simulink model "COM_ViconController_x4morf_quat_withRecov_posMod"  (Simulink 8.6)
settings: Solver=FixedStepDiscrete  StartTime=0.0  StopTime=inf  FixedStep=ComMinSampleTime  RelTol=1e-3
values from neighbouring files (symbols this model uses):
  a_PWM = (MaxThrottle-MinThrottle)/(omega_r_max-omega_r_min)    [RobotParameters.m]
  b_PWM = MinThrottle - a_PWM*omega_r_min    [RobotParameters.m]
  BiasAcc = [-0.0791 0.072 -0.1481]    [AccCalib_Transformation_X4morf_Robot.mat]
  ComMinSampleTime = 1/400    (= 0.0025)    [init_ViconController_x4morf_quat_withRecov_posMod.m]
  dc_close = 25    [RobotParameters.m]
  dc_open = 63    [RobotParameters.m]
  g = 9.81    [RobotParameters.m]    (also in init_ViconController_x4morf_quat_withRecov_posMod.m)
  gamma_max = 89    [RobotParameters.m]
  LandingHeight = 0.08    [init_ViconController_x4morf_quat_withRecov_posMod.m]
  m = 0.380    (= 0.38)    [RobotParameters.m]
  MaxThrottle = 2000    [RobotParameters.m]
  MinThrottle = 1200    [RobotParameters.m]
  PositionSecuMax = [5.5 ; 3 ; 4]    [RobotParameters.m]
  PositionSecuMin = [-0.5; -3; -0.07]    [RobotParameters.m]
  Tacc = [0.9812  -0.03737  -0.0078; 0.0368  0.9984  -0.0083; 0.0232  -0.0002  0.9804]    [AccCalib_Transformation_X4morf_Robot.mat]
  time_unfolding = 230e-3    (= 0.23)    [RobotParameters.m]
  Tmax = .1643    (= 0.1643)    [RobotParameters.m]
  Tmin = .0183    (= 0.0183)    [RobotParameters.m]
  TorquesSat = zeros(3,181)    [gen_iGamma.m]
  Ts_AttitudeLoop = 1/200    (= 0.005)    [init_ViconController_x4morf_quat_withRecov_posMod.m]
  Ts_PositionLoop = 1/100    (= 0.01)    [init_ViconController_x4morf_quat_withRecov_posMod.m]
  Velocity_0 = [Vx_0 Vy_0 Vz_0]    [RobotParameters.m]
undefined symbols (not defined in the file or in its folder): DiscIntNeverNeededParam, Gumstix, MPU6050, UAVstruct
undefined symbols (not defined in the file): AccMax, AccMaxScenario, AccMin, AccMinScenario, b_est0, PositionMax, PositionMin, SpeedMax, SpeedMaxScenario, SpeedMin, SpeedMinScenario, Ts_Wifi
libraries: simulink x40, simulink_extras x11
(part 2 of 3)

== system COM_ViconController_x4morf_quat_withRecov_posMod/GUMSTIX/Torques  Disturbances ==
  Torques : Inport
  Dist_Torques : Inport  Port=2
  " " : Constant  Value=[0 0 0]  OutDataTypeStr=Inherit: Inherit via back propagation
  Add : Sum
  Add1 : Sum
  Add2 : Sum
  Compare To Constant : simulink/Logic and Bit Operations/Compare To Constant  relop===  const=1  OutDataTypeStr=boolean
  Compare To Constant1 : simulink/Logic and Bit Operations/Compare To Constant  relop===  const=3  OutDataTypeStr=boolean
  Demux2 : Demux  Outputs=3
  Demux3 : Demux  Outputs=3
  Multiport Switch : MultiPortSwitch  DataPortForDefault=Additional data port
  Mux : Mux  Inputs=3
  Mux1 : Mux  Inputs=3
  Selector : Selector  InputPortWidth=5  IndexOptions=Index vector (dialog)  Indices=[1 2 3]  OutputSizes=1
  Selector2 : Selector  InputPortWidth=5  IndexOptions=Index vector (dialog)  Indices=4  OutputSizes=1
  Selector3 : Selector  InputPortWidth=5  IndexOptions=Index vector (dialog)  Indices=5  OutputSizes=1
  Triggered Subsystem : Subsystem  TreatAsAtomicUnit=on
  Triggered Subsystem1 : Subsystem  TreatAsAtomicUnit=on
  Torques_Out : Outport
  dist_torques_OUT : Outport  Port=2
  wires:
  Dist_Torques/1 -> Selector2/1, Selector3/1, Selector/1
  Selector/1 -> Triggered Subsystem1/1(TorquesDist Mag), Multiport Switch/3, Triggered Subsystem/1(TorquesDist Mag)
  Selector3/1 -> Mux1/3, Multiport Switch/1, Compare To Constant1/1, Compare To Constant/1
  Demux2/1 -> Add/1
  Demux2/2 -> Add1/1
  Demux2/3 -> Add2/1
  Add/1 -> Mux/1
  Add1/1 -> Mux/2
  Add2/1 -> Mux/3
  Demux3/2 -> Add1/2
  Demux3/1 -> Add/2
  Demux3/3 -> Add2/2
  Selector2/1 -> Mux1/2, Triggered Subsystem1/2(Dt), Triggered Subsystem/2(Dt)
  Torques/1 -> Demux2/1
  Mux/1 -> Torques_Out/1
  Compare To Constant/1 -> Triggered Subsystem/Enable
  Triggered Subsystem/1(DisturbTorques) -> Multiport Switch/2
  Multiport Switch/1 -> Demux3/1, Mux1/1
  " "/1 -> Multiport Switch/5
  Compare To Constant1/1 -> Triggered Subsystem1/Enable
  Triggered Subsystem1/1(DisturbTorques) -> Multiport Switch/4
  Mux1/1 -> dist_torques_OUT/1

== system COM_ViconController_x4morf_quat_withRecov_posMod/GUMSTIX/Torques saturation ==
  Torques : Inport
  gamma [deg] : Inport  Port=2
  Constant : Constant  Value=TorquesSat
  Convert : DataTypeConversion  RndMeth=Nearest
  Demux : Demux  Outputs=3
  Demux1 : Demux  Outputs=3
  Gain : Gain  Gain=-1
  Gain1 : Gain  Gain=-1
  Gain2 : Gain  Gain=-1
  MATLAB Function : MATLAB Function  TreatAsAtomicUnit=on
  Mux4 : Mux  Inputs=3
  Saturation Dynamic : simulink/Discontinuities/Saturation Dynamic  OutMin=[]  OutMax=[]  OutDataTypeStr=Inherit: Same as second input  OutDataType=fixdt(1, 16)  OutScaling=2^-10  DoSatur=off
  Saturation Dynamic1 : simulink/Discontinuities/Saturation Dynamic  OutMin=[]  OutMax=[]  OutDataTypeStr=Inherit: Same as second input  OutDataType=fixdt(1, 16)  OutScaling=2^-10  DoSatur=off
  Saturation Dynamic2 : simulink/Discontinuities/Saturation Dynamic  OutMin=[]  OutMax=[]  OutDataTypeStr=Inherit: Same as second input  OutDataType=fixdt(1, 16)  OutScaling=2^-10  DoSatur=off
  Torques_Sat : Outport
  Sats : Outport  Port=2
  wires:
  Mux4/1 -> Convert/1
  gamma [deg]/1 -> MATLAB Function/2(gamma)
  Constant/1 -> MATLAB Function/1(TorquesSat)
  Demux/1 -> Saturation Dynamic/2
  Demux/2 -> Saturation Dynamic1/2
  Demux/3 -> Saturation Dynamic2/2
  Saturation Dynamic/1 -> Mux4/1
  Saturation Dynamic1/1 -> Mux4/2
  Saturation Dynamic2/1 -> Mux4/3
  Torques/1 -> Demux/1
  Demux1/1 -> Gain/1, Saturation Dynamic/1
  Demux1/2 -> Gain1/1, Saturation Dynamic1/1
  Demux1/3 -> Gain2/1, Saturation Dynamic2/1
  Gain/1 -> Saturation Dynamic/3
  Gain1/1 -> Saturation Dynamic1/3
  Gain2/1 -> Saturation Dynamic2/3
  MATLAB Function/1(TSat) -> Sats/1, Demux1/1
  Convert/1 -> Torques_Sat/1

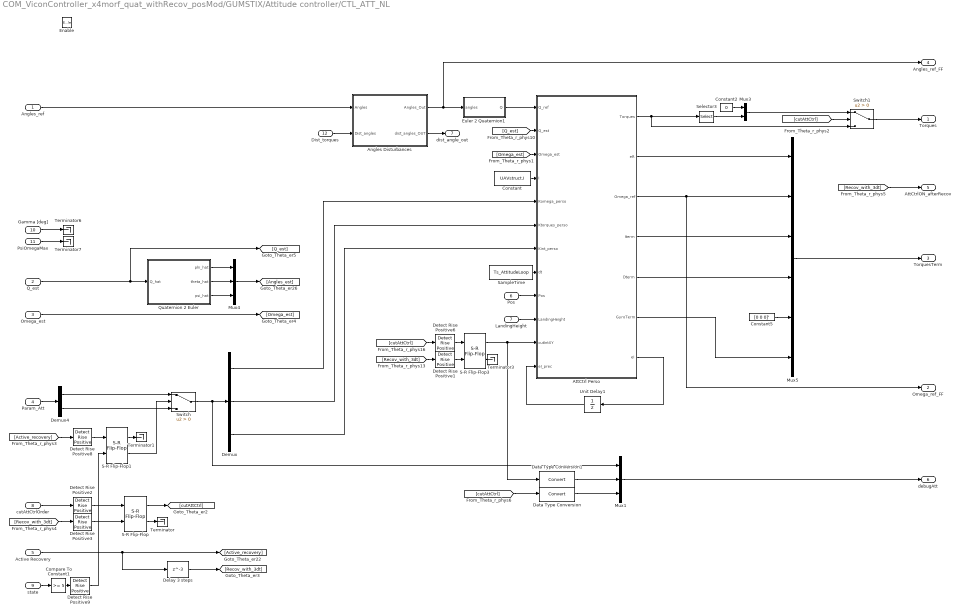
== system COM_ViconController_x4morf_quat_withRecov_posMod/GUMSTIX/Attitude controller/CTL_ATT_NL ==
  Angles_ref : Inport
  Q_est : Inport  Port=2
  Omega_est : Inport  Port=3
  Param_Att : Inport  Port=4
  Active Recovery : Inport  Port=5
  Pos : Inport  Port=6
  LandingHeight : Inport  Port=7
  cutAttCtrlOrder : Inport  Port=8
  state : Inport  Port=9
  Gamma [deg] : Inport  Port=10
  PsiOmegaMax : Inport  Port=11
  Dist_torques : Inport  Port=12
  Enable : EnablePort  StatesWhenEnabling=reset
  Angles Disturbances : Subsystem
  AttCtrl Perso : MATLAB Function  TreatAsAtomicUnit=on
  Compare To Constant1 : simulink/Logic and Bit Operations/Compare To Constant  relop=>=  const=5  OutDataTypeStr=boolean
  Constant : Constant  Value=UAVstruct.I  OutDataTypeStr=Inherit: Inherit via back propagation
  Constant2 : Constant  Value=0  OutDataTypeStr=Inherit: Inherit via back propagation
  Constant5 : Constant  Value=[0 0 0]'  OutDataTypeStr=Inherit: Inherit via back propagation
  Data Type Conversion : DataTypeConversion
  Data Type Conversion1 : DataTypeConversion
  Delay 3 steps : Delay  DelayLength=3  InitialCondition=0
  Demux : Demux  Outputs=[3 3 3]
  Demux4 : Demux  Outputs=2
  Detect Rise Positive{1..3,6,8..9} (6 alike) : simulink/Logic and Bit Operations/Detect Rise Positive  vinit=1  InputProcessing=Inherited  OutDataTypeStr=boolean
  Euler 2 Quaternion1 : MATLAB Function  TreatAsAtomicUnit=on
  Mux1 : Mux  Inputs=[9 1 1]
  Mux3 : Mux  Inputs=[1 2]
  Mux4 : Mux  Inputs=3
  Mux5 : Mux  Inputs=[3 3 3 3 3 3]
  Quaternion 2 Euler : MATLAB Function  TreatAsAtomicUnit=on
  S-R Flip-Flop : simulink_extras/Flip Flops/S-R Flip-Flop  initial_condition=0
  S-R Flip-Flop1 : simulink_extras/Flip Flops/S-R Flip-Flop  initial_condition=0
  S-R Flip-Flop3 : simulink_extras/Flip Flops/S-R Flip-Flop  initial_condition=0
  SampleTime : Constant  Value=Ts_AttitudeLoop  OutDataTypeStr=single  SampleTime=-1
  Selector3 : Selector  InputPortWidth=3  IndexOptions=Index vector (dialog)  Indices=[2 3]  OutputSizes=1
  Switch : Switch  Criteria=u2 > Threshold
  Switch1 : Switch  Criteria=u2 > Threshold
  Terminator{,1,3,6..7} (5 alike) : Terminator
  Unit Delay1 : UnitDelay  InitialCondition=single([0 0 0])  SampleTime=-1
  Torques : Outport  InitialOutput=[0; 0; 0]
  Omega_ref_FF : Outport  Port=2  InitialOutput=[0; 0; 0]
  TorquesTerm : Outport  Port=3  InitialOutput=zeros(18, 1)
  Angles_ref_FF : Outport  Port=4  InitialOutput=[0; 0; 0]
  AttCtrlON_afterRecov : Outport  Port=5  InitialOutput=0
  debugAtt : Outport  Port=6  InitialOutput=zeros(11,0)
  dist_angle_out : Outport  Port=7  InitialOutput=[0; 0; 0; 0; 0]
  wires:
  Constant2/1 -> Mux3/1
  Mux3/1 -> Switch1/1
  [cutAttCtrl] -> Switch1/2
  Active Recovery/1 -> Delay 3 steps/1, [Active_recovery]
  Delay 3 steps/1 -> [Recov_with_3dt]
  [Recov_with_3dt] -> Detect Rise Positive3/1
  [Recov_with_3dt] -> AttCtrlON_afterRecov/1
  Q_est/1 -> [Q_est], Quaternion 2 Euler/1(Q_hat)
  Omega_est/1 -> [Omega_est]
  Quaternion 2 Euler/1(phi_hat) -> Mux4/1
  Quaternion 2 Euler/2(theta_hat) -> Mux4/2
  Quaternion 2 Euler/3(psi_hat) -> Mux4/3
  Mux4/1 -> [Angles_est]
  cutAttCtrlOrder/1 -> Detect Rise Positive2/1
  S-R Flip-Flop/1 -> [cutAttCtrl]
  S-R Flip-Flop/2 -> Terminator/1
  Detect Rise Positive2/1 -> S-R Flip-Flop/1
  Detect Rise Positive3/1 -> S-R Flip-Flop/2
  Demux/1 -> AttCtrl Perso/5(Komega_perso)
  Demux/2 -> AttCtrl Perso/6(Ktorques_perso)
  Euler 2 Quaternion1/1(Q) -> AttCtrl Perso/1(Q_ref)
  AttCtrl Perso/1(Torques) -> Switch1/3, Selector3/1
  AttCtrl Perso/2(eR) -> Mux5/1
  AttCtrl Perso/6(GyroTerm) -> Mux5/6
  Mux5/1 -> TorquesTerm/1
  AttCtrl Perso/3(Omega_ref) -> Omega_ref_FF/1, Mux5/2
  AttCtrl Perso/7(eI) -> Unit Delay1/1
  Unit Delay1/1 -> AttCtrl Perso/12(eI_prec)
  AttCtrl Perso/4(Iterm) -> Mux5/3
  Demux/3 -> AttCtrl Perso/7(Kint_perso)
  Switch1/1 -> Torques/1
  state/1 -> Compare To Constant1/1
  AttCtrl Perso/5(Dterm) -> Mux5/4
  S-R Flip-Flop3/1 -> Data Type Conversion1/1, AttCtrl Perso/11(cutIntXY)
  S-R Flip-Flop3/2 -> Terminator3/1
  [cutAttCtrl] -> Detect Rise Positive6/1
  Detect Rise Positive6/1 -> S-R Flip-Flop3/1
  Detect Rise Positive1/1 -> S-R Flip-Flop3/2
  Gamma [deg]/1 -> Terminator6/1
  PsiOmegaMax/1 -> Terminator7/1
  Constant5/1 -> Mux5/5
  [Recov_with_3dt] -> Detect Rise Positive1/1
  Constant/1 -> AttCtrl Perso/4(I)
  SampleTime/1 -> AttCtrl Perso/8(dt)
  Pos/1 -> AttCtrl Perso/9(Pos)
  LandingHeight/1 -> AttCtrl Perso/10(LandingHeight)
  [Omega_est] -> AttCtrl Perso/3(Omega_est)
  Param_Att/1 -> Demux4/1
  Demux4/1 -> Switch/1
  Demux4/2 -> Switch/3
  Switch/1 -> Mux1/1, Demux/1
  [Active_recovery] -> Detect Rise Positive8/1
  Detect Rise Positive8/1 -> S-R Flip-Flop1/1
  S-R Flip-Flop1/1 -> Terminator1/1
  S-R Flip-Flop1/2 -> Switch/2
  Compare To Constant1/1 -> Detect Rise Positive9/1
  Detect Rise Positive9/1 -> S-R Flip-Flop1/2
  [cutAttCtrl] -> Data Type Conversion/1
  Mux1/1 -> debugAtt/1
  Data Type Conversion/1 -> Mux1/3
  Data Type Conversion1/1 -> Mux1/2
  Angles Disturbances/1(Angles_Out) -> Angles_ref_FF/1, Euler 2 Quaternion1/1(angles)
  Angles Disturbances/2(dist_angles_OUT) -> dist_angle_out/1
  Dist_torques/1 -> Angles Disturbances/2(Dist_angles)
  [Q_est] -> AttCtrl Perso/2(Q_est)
  Angles_ref/1 -> Angles Disturbances/1(Angles)
  Selector3/1 -> Mux3/2

== system COM_ViconController_x4morf_quat_withRecov_posMod/GUMSTIX/Control Mix/Control_mix ==
  Thrust : Inport
  Torques : Inport  Port=2
  gamma [deg] : Inport  Port=3
  Constant : Constant  Value=UAVstruct.iGamma  OutDataTypeStr=Inherit: Inherit via back propagation
  Demux : Demux
  Mixage : MATLAB Function  TreatAsAtomicUnit=on
  Mux1 : Mux  Inputs=2
  Rate Transition : RateTransition
  Saturation1 : Saturate  UpperLimit=inf  LowerLimit=0
  Sqrt1 : Sqrt  SaturateOnIntegerOverflow=on
  omega_r1_ref : Outport
  omega_r2_ref : Outport  Port=2
  omega_r3_ref : Outport  Port=3
  omega_r4_ref : Outport  Port=4
  wires:
  Demux/1 -> omega_r1_ref/1
  Demux/2 -> omega_r2_ref/1
  Demux/3 -> omega_r3_ref/1
  Demux/4 -> omega_r4_ref/1
  Sqrt1/1 -> Rate Transition/1
  Rate Transition/1 -> Demux/1
  Thrust/1 -> Mux1/1
  Torques/1 -> Mux1/2
  Mixage/1(omega2) -> Saturation1/1
  Saturation1/1 -> Sqrt1/1
  gamma [deg]/1 -> Mixage/3(gamma)
  Mux1/1 -> Mixage/2(ThrustTorques)
  Constant/1 -> Mixage/1(iGamma)

== system COM_ViconController_x4morf_quat_withRecov_posMod/GUMSTIX/Control Mix/Omega_ref 2 PWM_ref ==
  Omega_ref : Inport
  Bias : Bias  Bias=b_PWM
  Gain : Gain  Gain=a_PWM
  PWM_ref : Outport
  wires:
  Gain/1 -> Bias/1
  Bias/1 -> PWM_ref/1
  Omega_ref/1 -> Gain/1

== system COM_ViconController_x4morf_quat_withRecov_posMod/GUMSTIX/ESTIMATOR/Complementary Filter Quaternion gyro, acc, vicon GUMSTIX ==
  gyro : Inport
  acc : Inport  Port=2
  Vicon_Quaternion : Inport  Port=3
  k_a : Inport  Port=4
  k_v : Inport  Port=5
  k_b : Inport  Port=6
  Attitude_Est : MATLAB Function  TreatAsAtomicUnit=on
  Bias : Delay  DelayLength=1  InitialCondition=b0_param  SampleTime=Ts_param
  Constant1 : Constant  Value=Ts_param  OutDataTypeStr=Inherit: Inherit via back propagation
  Constant7 : Constant  Value=acc_ref_param  VectorParams1D=off  OutDataTypeStr=Inherit: Inherit via back propagation
  Quaternion : Delay  DelayLength=1  InitialCondition=Q0_param  SampleTime=Ts_param
  b_hat [rad/sec] : Outport
  Q_hat : Outport  Port=2
  Omega_hat [rad/sec] : Outport  Port=3
  wires:
  Attitude_Est/1(Q_hat) -> Q_hat/1, Quaternion/1
  Attitude_Est/2(b_hat) -> Bias/1, b_hat [rad/sec]/1
  Constant1/1 -> Attitude_Est/6(dt)
  Bias/1 -> Attitude_Est/2(b_hat_prec)
  Quaternion/1 -> Attitude_Est/1(Q_hat_prec)
  Attitude_Est/3(Omega_hat) -> Omega_hat [rad/sec]/1
  acc/1 -> Attitude_Est/4(acc_imu)
  gyro/1 -> Attitude_Est/3(gyro_imu)
  Constant7/1 -> Attitude_Est/10(acc_ref)
  Vicon_Quaternion/1 -> Attitude_Est/5(Q_Vicon)
  k_a/1 -> Attitude_Est/7(k_a)
  k_v/1 -> Attitude_Est/8(k_v)
  k_b/1 -> Attitude_Est/9(k_b)

== system COM_ViconController_x4morf_quat_withRecov_posMod/GUMSTIX/ESTIMATOR/Unbias Sensors ==
  Sensors : Inport
  Bias : Bias  Bias=-BiasAcc
  Constant : Constant  Value=single(Tacc)
  Demux2 : Demux  Outputs=[3 3]
  Product : Product  Multiplication=Matrix(*)  RndMeth=Zero
  int16_2_g : Gain  Gain=MPU6050.acc.int16_2_g  OutDataTypeStr=Inherit: Same as input
  int16_2_rad : Gain  Gain=MPU6050.gyr.int16_2_rad  OutDataTypeStr=Inherit: Same as input
  RAW_Gyro : Outport
  Unbiased_Acc : Outport  Port=2
  RAW_Acc : Outport  Port=3
  wires:
  Sensors/1 -> Demux2/1
  int16_2_g/1 -> RAW_Acc/1, Bias/1
  Demux2/1 -> int16_2_rad/1
  int16_2_rad/1 -> RAW_Gyro/1
  Demux2/2 -> int16_2_g/1
  Bias/1 -> Product/2
  Constant/1 -> Product/1
  Product/1 -> Unbiased_Acc/1

== system COM_ViconController_x4morf_quat_withRecov_posMod/GUMSTIX/Manual_Controller/RX Angles Ref  Generator ==
  Roll_RX : Inport
  Pitch_RX : Inport  Port=2
  Yaw_RX : Inport  Port=3
  Throttle_RX : Inport  Port=4
  Rescale Pitch : Subsystem  mask{MinInput=1000, MaxInput=2000, DeadZone=10, MinOutput=-20*pi/180, MaxOutput=20*pi/180, G_Scale=0, BiasScale=0}
      mask prompts: MinInput "Minimum Input"; MaxInput "Maximum Input"; DeadZone "Dead Zone"; MinOutput "Minimum Output"; MaxOutput "Maximum Output"; BiasScale "Bias_Scale"
      mask init:
      | Gscale = (MaxOutput-MinOutput)/(MaxInput-MinInput-2*DeadZone);
      | Bias_Scale = MinInput+(MaxInput-MinInput)/2;
  Rescale Roll : Subsystem  mask{MinInput=1000, MaxInput=2000, DeadZone=10, MinOutput=-20*pi/180, MaxOutput=20*pi/180, G_Scale=0, BiasScale=0}
      mask prompts: MinInput "Minimum Input"; MaxInput "Maximum Input"; DeadZone "Dead Zone"; MinOutput "Minimum Output"; MaxOutput "Maximum Output"; BiasScale "Bias_Scale"
      mask init:
      | Gscale = (MaxOutput-MinOutput)/(MaxInput-MinInput-2*DeadZone);
      | Bias_Scale = MinInput+(MaxInput-MinInput)/2;
  Rescale Yaw : Subsystem  mask{MinInput=1000, MaxInput=2000, DeadZone=10, MinOutput=-30*pi/180, MaxOutput=30*pi/180, G_Scale=0, BiasScale=0}
      mask prompts: MinInput "Minimum Input"; MaxInput "Maximum Input"; DeadZone "Dead Zone"; MinOutput "Minimum Output"; MaxOutput "Maximum Output"; BiasScale "Bias_Scale"
      mask init:
      | Gscale = (MaxOutput-MinOutput)/(MaxInput-MinInput-2*DeadZone);
      | Bias_Scale = MinInput+(MaxInput-MinInput)/2;
  Rescale2 Throttle : Subsystem  mask{MinInput=1000, MaxInput=2000, MinOutput=0*m*g, MaxOutput=1.3*m*g, G_Scale=0}
      mask prompts: MinInput "Minimum Input"; MaxInput "Maximum Input"; MinOutput "Minimum Output"; MaxOutput "Maximum Output"
      mask init:
      | Gscale = (MaxOutput-MinOutput)/(MaxInput-MinInput);
  Roll_ref : Outport
  Pitch_ref : Outport  Port=2
  Yaw_ref : Outport  Port=3
  Throttle_ref : Outport  Port=4
  wires:
  Roll_RX/1 -> Rescale Roll/1(In)
  Pitch_RX/1 -> Rescale Pitch/1(In)
  Yaw_RX/1 -> Rescale Yaw/1(In)
  Rescale Roll/1(Out) -> Roll_ref/1
  Rescale Pitch/1(Out) -> Pitch_ref/1
  Rescale Yaw/1(Out) -> Yaw_ref/1
  Throttle_RX/1 -> Rescale2 Throttle/1(In)
  Rescale2 Throttle/1(Out) -> Throttle_ref/1

== system COM_ViconController_x4morf_quat_withRecov_posMod/GUMSTIX/PWM/deg convert/PWM to gamma ==
  PWM [in %] : Inport
  Bias : Bias  Bias=-dc_open
  Gain : Gain  Gain=gamma_max/(dc_close-dc_open)
  Saturation : Saturate  UpperLimit=gamma_max  LowerLimit=0
  gamma [deg] : Outport
  wires:
  PWM [in %]/1 -> Bias/1
  Gain/1 -> Saturation/1
  Saturation/1 -> gamma [deg]/1
  Bias/1 -> Gain/1

== system COM_ViconController_x4morf_quat_withRecov_posMod/GUMSTIX/PWM/deg convert/gamma to PWM ==
  gamma [deg] : Inport
  Bias : Bias  Bias=dc_open
  Gain : Gain  Gain=(dc_close-dc_open)/gamma_max
  Saturation : Saturate  UpperLimit=max(dc_close,dc_open)  LowerLimit=min(dc_close,dc_open)
  PWM [in %] : Outport
  wires:
  gamma [deg]/1 -> Gain/1
  Bias/1 -> Saturation/1
  Gain/1 -> Bias/1
  Saturation/1 -> PWM [in %]/1

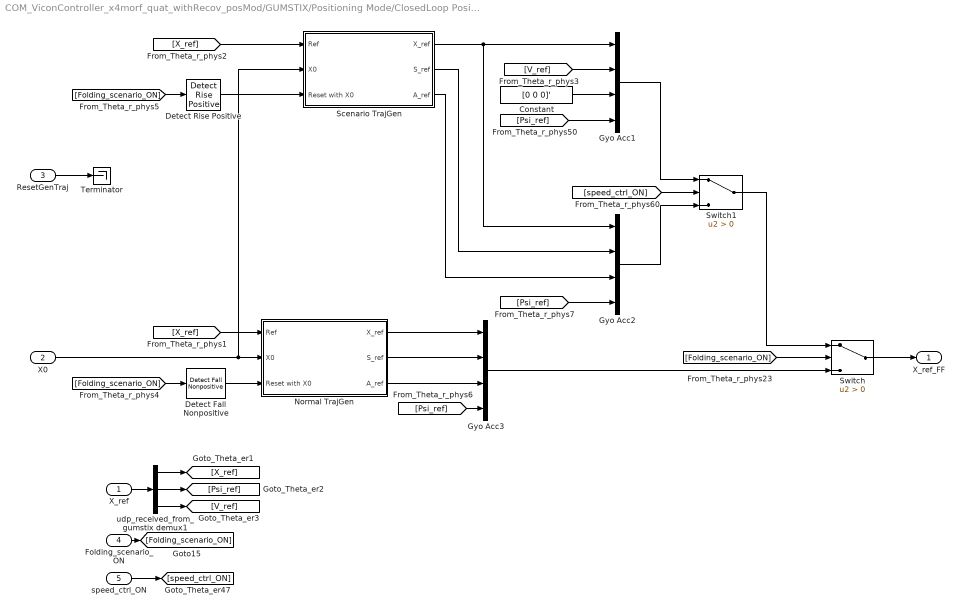
== system COM_ViconController_x4morf_quat_withRecov_posMod/GUMSTIX/Positioning Mode/ClosedLoop Position SetPoint Generator ==
  X_ref : Inport
  X0 : Inport  Port=2
  ResetGenTraj : Inport  Port=3
  Folding_scenario_ON : Inport  Port=4
  speed_ctrl_ON : Inport  Port=5
  Constant : Constant  Value=[0 0 0]'  OutDataTypeStr=Inherit: Inherit via back propagation
  Detect Fall Nonpositive : simulink/Logic and Bit Operations/Detect Fall Nonpositive  vinit=1  InputProcessing=Inherited  OutDataTypeStr=boolean
  Detect Rise Positive : simulink/Logic and Bit Operations/Detect Rise Positive  vinit=1  InputProcessing=Inherited  OutDataTypeStr=boolean
  Gyo Acc1 : Mux
  Gyo Acc2 : Mux
  Gyo Acc3 : Mux
  Normal TrajGen : Subsystem  mask{Tau=[3/6 3/6 5/6]', Ts_Filter=Ts_PositionLoop, Xmax=PositionMax, Xmin=PositionMin, Smax=SpeedMax, Smin=SpeedMin, Amax=AccMax, Amin=AccMin}
      mask prompts: Ts_Filter "Ts"; Xmax "Pos max"; Xmin "Pos min"; Smax "Speed max"; Smin "Speed min"; Amax "Acc max"; Amin "Acc min"
  Scenario TrajGen : Subsystem  mask{Tau=[3/6 3/6 5/6]', Ts_Filter=Ts_PositionLoop, Xmax=PositionMax, Xmin=PositionMin, Smax=SpeedMaxScenario, Smin=SpeedMinScenario, Amax=AccMaxScenario, Amin=AccMinScenario}
      mask prompts: Ts_Filter "Ts"; Xmax "Pos max"; Xmin "Pos min"; Smax "Speed max"; Smin "Speed min"; Amax "Acc max"; Amin "Acc min"
  Switch : Switch  Criteria=u2 > Threshold
  Switch1 : Switch  Criteria=u2 > Threshold
  Terminator : Terminator
  udp_received_from_gumstix demux1 : Demux  Outputs=[3 1 3]
  X_ref_FF : Outport
  wires:
  [X_ref] -> Normal TrajGen/1(Ref)
  udp_received_from_gumstix demux1/1 -> [X_ref]
  udp_received_from_gumstix demux1/2 -> [Psi_ref]
  X_ref/1 -> udp_received_from_gumstix demux1/1
  [Psi_ref] -> Gyo Acc1/4
  Normal TrajGen/1(X_ref) -> Gyo Acc3/1
  Normal TrajGen/2(S_ref) -> Gyo Acc3/2
  Normal TrajGen/3(A_ref) -> Gyo Acc3/3
  Folding_scenario_ON/1 -> [Folding_scenario_ON]
  [Folding_scenario_ON] -> Switch/2
  Switch/1 -> X_ref_FF/1
  Gyo Acc3/1 -> Switch/3
  ResetGenTraj/1 -> Terminator/1
  [Folding_scenario_ON] -> Detect Fall Nonpositive/1
  Detect Fall Nonpositive/1 -> Normal TrajGen/3(Reset with X0)
  [V_ref] -> Gyo Acc1/2
  Constant/1 -> Gyo Acc1/3
  X0/1 -> Scenario TrajGen/2(X0), Normal TrajGen/2(X0)
  udp_received_from_gumstix demux1/3 -> [V_ref]
  [X_ref] -> Scenario TrajGen/1(Ref)
  Scenario TrajGen/1(X_ref) -> Gyo Acc2/1, Gyo Acc1/1
  [Folding_scenario_ON] -> Detect Rise Positive/1
  Detect Rise Positive/1 -> Scenario TrajGen/3(Reset with X0)
  Scenario TrajGen/2(S_ref) -> Gyo Acc2/2
  Scenario TrajGen/3(A_ref) -> Gyo Acc2/3
  speed_ctrl_ON/1 -> [speed_ctrl_ON]
  [speed_ctrl_ON] -> Switch1/2
  [Psi_ref] -> Gyo Acc3/4
  Switch1/1 -> Switch/1
  Gyo Acc1/1 -> Switch1/1
  Gyo Acc2/1 -> Switch1/3
  [Psi_ref] -> Gyo Acc2/4

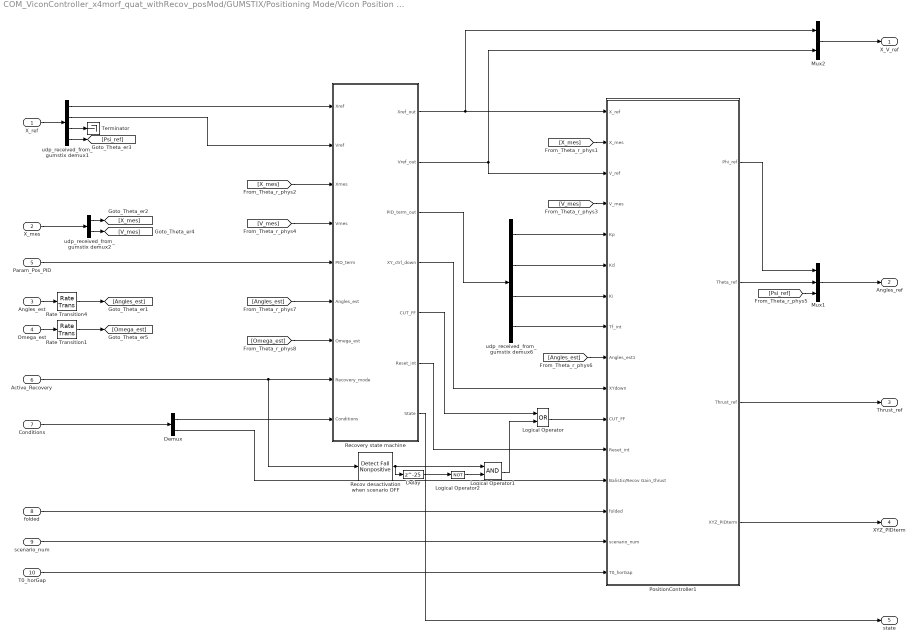
== system COM_ViconController_x4morf_quat_withRecov_posMod/GUMSTIX/Positioning Mode/Vicon Position  Controller ==
  X_ref : Inport
  X_mes : Inport  Port=2
  Angles_est : Inport  Port=3
  Omega_est : Inport  Port=4
  Param_Pos_PID : Inport  Port=5
  Active_Recovery : Inport  Port=6
  Conditions : Inport  Port=7
  folded : Inport  Port=8
  scenario_num : Inport  Port=9
  T0_horGap : Inport  Port=10
  Delay : Delay  DelayLength=25  InitialCondition=0
  Demux : Demux  Outputs=[4 2]
  Logical Operator : Logic  Operator=OR  AllPortsSameDT=off  OutDataTypeStr=boolean
  Logical Operator1 : Logic  AllPortsSameDT=off  OutDataTypeStr=boolean
  Logical Operator2 : Logic  Operator=NOT  AllPortsSameDT=off  OutDataTypeStr=boolean
  Mux1 : Mux  Inputs=[1 1 1]
  Mux2 : Mux  Inputs=2
  PositionController1 : Subsystem
  Rate Transition1 : RateTransition  OutPortSampleTime=Ts_PositionLoop
  Rate Transition4 : RateTransition  OutPortSampleTime=Ts_PositionLoop
  Recov desactivation when scenario OFF : simulink/Logic and Bit Operations/Detect Fall Nonpositive  vinit=1  InputProcessing=Inherited  OutDataTypeStr=boolean
  Recovery state machine : Subsystem
  Terminator : Terminator
  udp_received_from_gumstix demux1 : Demux  Outputs=[3 3 3 1]
  udp_received_from_gumstix demux2 : Demux  Outputs=[3 3]
  udp_received_from_gumstix demux6 : Demux  Outputs=[3 3 3 3]
  X_V_ref : Outport  InitialOutput=eye(3, 3)
  Angles_ref : Outport  Port=2  InitialOutput=eye(3, 3)
  Thrust_ref : Outport  Port=3  InitialOutput=0
  XYZ_PIDterm : Outport  Port=4  InitialOutput=0
  state : Outport  Port=5  InitialOutput=0
  wires:
  Mux1/1 -> Angles_ref/1
  PositionController1/3(Thrust_ref) -> Thrust_ref/1
  X_ref/1 -> udp_received_from_gumstix demux1/1
  Angles_est/1 -> Rate Transition4/1
  udp_received_from_gumstix demux2/1 -> [X_mes]
  udp_received_from_gumstix demux2/2 -> [V_mes]
  udp_received_from_gumstix demux1/4 -> [Psi_ref]
  PositionController1/1(Phi_ref) -> Mux1/1
  PositionController1/2(Theta_ref) -> Mux1/2
  [Psi_ref] -> Mux1/3
  udp_received_from_gumstix demux6/1 -> PositionController1/5(Kp)
  udp_received_from_gumstix demux6/2 -> PositionController1/6(Kd)
  udp_received_from_gumstix demux6/3 -> PositionController1/7(Ki)
  udp_received_from_gumstix demux6/4 -> PositionController1/8(Tf_int)
  udp_received_from_gumstix demux1/3 -> Terminator/1
  Recovery state machine/4(XY_ctrl_down) -> PositionController1/10(XYdown)
  udp_received_from_gumstix demux1/1 -> Recovery state machine/1(Xref)
  [X_mes] -> Recovery state machine/3(Xmes)
  [V_mes] -> Recovery state machine/4(Vmes)
  Param_Pos_PID/1 -> Recovery state machine/5(PID_term)
  Active_Recovery/1 -> Recov desactivation when scenario OFF/1, Recovery state machine/8(Recovery_mode)
  Recovery state machine/3(PID_term_out) -> udp_received_from_gumstix demux6/1
  Recovery state machine/2(Vref_out) -> PositionController1/3(V_ref), Mux2/2
  Recovery state machine/1(Xref_out) -> Mux2/1, PositionController1/1(X_ref)
  udp_received_from_gumstix demux1/2 -> Recovery state machine/2(Vref)
  X_mes/1 -> udp_received_from_gumstix demux2/1
  [X_mes] -> PositionController1/2(X_mes)
  [V_mes] -> PositionController1/4(V_mes)
  Rate Transition4/1 -> [Angles_est]
  [Angles_est] -> PositionController1/9(Angles_est1)
  [Angles_est] -> Recovery state machine/6(Angles_est)
  Omega_est/1 -> Rate Transition1/1
  Rate Transition1/1 -> [Omega_est]
  [Omega_est] -> Recovery state machine/7(Omega_est)
  Recovery state machine/6(Reset_int) -> PositionController1/12(Reset_int)
  Mux2/1 -> X_V_ref/1
  PositionController1/4(XYZ_PIDterm) -> XYZ_PIDterm/1
  Recovery state machine/7(State) -> state/1
  Demux/1 -> Recovery state machine/9(Conditions)
  Conditions/1 -> Demux/1
  Demux/2 -> PositionController1/13(Balistic/Recov Gain_thrust)
  folded/1 -> PositionController1/14(folded)
  Logical Operator/1 -> PositionController1/11(CUT_FF)
  Recovery state machine/5(CUT_FF) -> Logical Operator/1
  Logical Operator1/1 -> Logical Operator/2
  Delay/1 -> Logical Operator2/1
  Recov desactivation when scenario OFF/1 -> Delay/1, Logical Operator1/1
  Logical Operator2/1 -> Logical Operator1/2
  scenario_num/1 -> PositionController1/15(scenario_num)
  T0_horGap/1 -> PositionController1/16(T0_horGap)

== system COM_ViconController_x4morf_quat_withRecov_posMod/GUMSTIX/Torques  Disturbances/Triggered Subsystem ==
  TorquesDist Mag : Inport
  Dt : Inport  Port=2
  Enable : EnablePort  StatesWhenEnabling=reset
  Constant : Constant  OutDataTypeStr=single
  Discrete-Time Integrator : DiscreteIntegrator  SampleTime=-1  ICPrevOutput=DiscIntNeverNeededParam  ICPrevScaledInput=DiscIntNeverNeededParam
  MATLAB Function : MATLAB Function  TreatAsAtomicUnit=on
  DisturbTorques : Outport  InitialOutput=[0 0 0]
  wires:
  TorquesDist Mag/1 -> MATLAB Function/1(TorquesDistMag)
  Constant/1 -> Discrete-Time Integrator/1
  Discrete-Time Integrator/1 -> MATLAB Function/2(Time)
  Dt/1 -> MATLAB Function/3(Dt)
  MATLAB Function/1(TorquesDist) -> DisturbTorques/1

== system COM_ViconController_x4morf_quat_withRecov_posMod/GUMSTIX/Torques  Disturbances/Triggered Subsystem1 ==
  TorquesDist Mag : Inport
  Dt : Inport  Port=2
  Enable : EnablePort  StatesWhenEnabling=reset
  Constant : Constant  OutDataTypeStr=single
  Discrete-Time Integrator : DiscreteIntegrator  SampleTime=-1  ICPrevOutput=DiscIntNeverNeededParam  ICPrevScaledInput=DiscIntNeverNeededParam
  MATLAB Function : MATLAB Function  TreatAsAtomicUnit=on
  DisturbTorques : Outport  InitialOutput=[0 0 0]
  wires:
  TorquesDist Mag/1 -> MATLAB Function/1(TorquesDistMag)
  Constant/1 -> Discrete-Time Integrator/1
  Discrete-Time Integrator/1 -> MATLAB Function/2(Time)
  Dt/1 -> MATLAB Function/3(Dt)
  MATLAB Function/1(TorquesDist) -> DisturbTorques/1

== system COM_ViconController_x4morf_quat_withRecov_posMod/GUMSTIX/Attitude controller/CTL_ATT_NL/Angles Disturbances ==
  Angles : Inport
  Dist_angles : Inport  Port=2
  Add : Sum
  Add1 : Sum
  Add2 : Sum
  Compare To Constant : simulink/Logic and Bit Operations/Compare To Constant  relop===  const=4  OutDataTypeStr=boolean
  Demux2 : Demux  Outputs=3
  Demux3 : Demux  Outputs=3
  Mux : Mux  Inputs=3
  Mux1 : Mux  Inputs=3
  Selector : Selector  InputPortWidth=5  IndexOptions=Index vector (dialog)  Indices=[1 2 3]  OutputSizes=1
  Selector2 : Selector  InputPortWidth=5  IndexOptions=Index vector (dialog)  Indices=4  OutputSizes=1
  Selector3 : Selector  InputPortWidth=5  IndexOptions=Index vector (dialog)  Indices=5  OutputSizes=1
  Triggered Subsystem : Subsystem  TreatAsAtomicUnit=on
  Angles_Out : Outport
  dist_angles_OUT : Outport  Port=2
  wires:
  Dist_angles/1 -> Selector2/1, Selector3/1, Selector/1
  Selector/1 -> Triggered Subsystem/1(AnglesDist Mag)
  Selector3/1 -> Mux1/3, Compare To Constant/1
  Demux2/1 -> Add/1
  Demux2/2 -> Add1/1
  Demux2/3 -> Add2/1
  Add/1 -> Mux/1
  Add1/1 -> Mux/2
  Add2/1 -> Mux/3
  Demux3/2 -> Add1/2
  Demux3/1 -> Add/2
  Demux3/3 -> Add2/2
  Selector2/1 -> Mux1/2, Triggered Subsystem/2(Dt)
  Angles/1 -> Demux2/1
  Mux/1 -> Angles_Out/1
  Compare To Constant/1 -> Triggered Subsystem/Enable
  Triggered Subsystem/1(DisturbAngles) -> Demux3/1, Mux1/1
  Mux1/1 -> dist_angles_OUT/1

== system COM_ViconController_x4morf_quat_withRecov_posMod/GUMSTIX/Manual_Controller/RX Angles Ref  Generator/Rescale Pitch ==
  In : Inport
  Bias : Bias  Bias=-Bias_Scale
  Dead Zone : DeadZone  LowerValue=-DeadZone  UpperValue=DeadZone  SaturateOnIntegerOverflow=on
  Gain : Gain  Gain=Gscale
  Saturation : Saturate  UpperLimit=MaxOutput  LowerLimit=MinOutput
  Out : Outport
  wires:
  Bias/1 -> Dead Zone/1
  In/1 -> Bias/1
  Dead Zone/1 -> Gain/1
  Saturation/1 -> Out/1
  Gain/1 -> Saturation/1

== system COM_ViconController_x4morf_quat_withRecov_posMod/GUMSTIX/Manual_Controller/RX Angles Ref  Generator/Rescale Roll ==
  In : Inport
  Bias : Bias  Bias=-Bias_Scale
  Dead Zone : DeadZone  LowerValue=-DeadZone  UpperValue=DeadZone  SaturateOnIntegerOverflow=on
  Gain : Gain  Gain=Gscale
  Saturation : Saturate  UpperLimit=MaxOutput  LowerLimit=MinOutput
  Out : Outport
  wires:
  Gain/1 -> Saturation/1
  Saturation/1 -> Out/1
  Dead Zone/1 -> Gain/1
  In/1 -> Bias/1
  Bias/1 -> Dead Zone/1

== system COM_ViconController_x4morf_quat_withRecov_posMod/GUMSTIX/Manual_Controller/RX Angles Ref  Generator/Rescale Yaw ==
  In : Inport
  Bias : Bias  Bias=-Bias_Scale
  Dead Zone : DeadZone  LowerValue=-DeadZone  UpperValue=DeadZone  SaturateOnIntegerOverflow=on
  Gain : Gain  Gain=Gscale
  Saturation : Saturate  UpperLimit=MaxOutput  LowerLimit=MinOutput
  Out : Outport
  wires:
  Gain/1 -> Saturation/1
  Saturation/1 -> Out/1
  Dead Zone/1 -> Gain/1
  In/1 -> Bias/1
  Bias/1 -> Dead Zone/1

== system COM_ViconController_x4morf_quat_withRecov_posMod/GUMSTIX/Manual_Controller/RX Angles Ref  Generator/Rescale2 Throttle ==
  In : Inport
  Bias : Bias  Bias=-MinInput
  Gain : Gain  Gain=Gscale
  Saturation : Saturate  UpperLimit=MaxOutput  LowerLimit=MinOutput
  Out : Outport
  wires:
  Bias/1 -> Gain/1
  In/1 -> Bias/1
  Saturation/1 -> Out/1
  Gain/1 -> Saturation/1

== system COM_ViconController_x4morf_quat_withRecov_posMod/GUMSTIX/Positioning Mode/ClosedLoop Position SetPoint Generator/Normal TrajGen ==
  Ref : Inport
  X0 : Inport  Port=2
  Reset with X0 : Inport  Port=3
  Add : Sum  Inputs=+-
  Gain : Gain  Gain=2*Tau.^2
  Gain1 : Gain  Gain=3*Tau
  Gain3 : Gain  Gain=1./Tau.^3
  Rate Transition3 : RateTransition  Deterministic=off
  Saturation : Saturate  UpperLimit=Xmax  LowerLimit=Xmin
  Selector1 : Selector  InputPortWidth=6  IndexOptions=Index vector (dialog)  Indices=[1 2 3]  OutputSizes=1
  Selector2 : Selector  InputPortWidth=6  IndexOptions=Index vector (dialog)  Indices=[4 5 6]  OutputSizes=1
  Sum : Sum  Inputs=+|+|+
  dA : DiscreteIntegrator  ExternalReset=rising  SampleTime=Ts_Filter  LimitOutput=on  UpperSaturationLimit=Amax  LowerSaturationLimit=Amin  ICPrevOutput=DiscIntNeverNeededParam  ICPrevScaledInput=DiscIntNeverNeededParam
  dV : DiscreteIntegrator  ExternalReset=rising  InitialConditionSource=external  SampleTime=Ts_Filter  LimitOutput=on  UpperSaturationLimit=Smax  LowerSaturationLimit=Smin  ICPrevOutput=DiscIntNeverNeededParam  ICPrevScaledInput=DiscIntNeverNeededParam
  dX : DiscreteIntegrator  ExternalReset=rising  InitialConditionSource=external  SampleTime=Ts_Filter  LimitOutput=on  UpperSaturationLimit=Xmax  LowerSaturationLimit=Xmin  ICPrevOutput=DiscIntNeverNeededParam  ICPrevScaledInput=DiscIntNeverNeededParam
  X_ref : Outport
  S_ref : Outport  Port=2
  A_ref : Outport  Port=3
  wires:
  Saturation/1 -> Add/1
  Gain3/1 -> dA/1
  Gain/1 -> Sum/1
  Gain1/1 -> Sum/2
  Add/1 -> Gain3/1
  dV/1 -> S_ref/1, Gain1/1, dX/1
  dA/1 -> A_ref/1, Gain/1, dV/1
  dX/1 -> Sum/3, X_ref/1
  Ref/1 -> Saturation/1
  Reset with X0/1 -> Rate Transition3/1
  Sum/1 -> Add/2
  X0/1 -> Selector1/1, Selector2/1
  Selector1/1 -> dX/3
  Selector2/1 -> dV/3
  Rate Transition3/1 -> dV/2, dX/2, dA/2

== system COM_ViconController_x4morf_quat_withRecov_posMod/GUMSTIX/Positioning Mode/ClosedLoop Position SetPoint Generator/Scenario TrajGen ==
  Ref : Inport
  X0 : Inport  Port=2
  Reset with X0 : Inport  Port=3
  Add : Sum  Inputs=+-
  Gain : Gain  Gain=2*Tau.^2
  Gain1 : Gain  Gain=3*Tau
  Gain3 : Gain  Gain=1./Tau.^3
  Rate Transition3 : RateTransition  Deterministic=off
  Saturation : Saturate  UpperLimit=Xmax  LowerLimit=Xmin
  Selector1 : Selector  InputPortWidth=6  IndexOptions=Index vector (dialog)  Indices=[1 2 3]  OutputSizes=1
  Selector2 : Selector  InputPortWidth=6  IndexOptions=Index vector (dialog)  Indices=[4 5 6]  OutputSizes=1
  Sum : Sum  Inputs=+|+|+
  dA : DiscreteIntegrator  ExternalReset=rising  SampleTime=Ts_Filter  LimitOutput=on  UpperSaturationLimit=Amax  LowerSaturationLimit=Amin  ICPrevOutput=DiscIntNeverNeededParam  ICPrevScaledInput=DiscIntNeverNeededParam
  dV : DiscreteIntegrator  ExternalReset=rising  InitialConditionSource=external  SampleTime=Ts_Filter  LimitOutput=on  UpperSaturationLimit=Smax  LowerSaturationLimit=Smin  ICPrevOutput=DiscIntNeverNeededParam  ICPrevScaledInput=DiscIntNeverNeededParam
  dX : DiscreteIntegrator  ExternalReset=rising  InitialConditionSource=external  SampleTime=Ts_Filter  LimitOutput=on  UpperSaturationLimit=Xmax  LowerSaturationLimit=Xmin  ICPrevOutput=DiscIntNeverNeededParam  ICPrevScaledInput=DiscIntNeverNeededParam
  X_ref : Outport
  S_ref : Outport  Port=2
  A_ref : Outport  Port=3
  wires:
  Saturation/1 -> Add/1
  Gain3/1 -> dA/1
  Gain/1 -> Sum/1
  Gain1/1 -> Sum/2
  Add/1 -> Gain3/1
  dV/1 -> S_ref/1, Gain1/1, dX/1
  dA/1 -> A_ref/1, Gain/1, dV/1
  dX/1 -> Sum/3, X_ref/1
  Ref/1 -> Saturation/1
  Reset with X0/1 -> Rate Transition3/1
  Sum/1 -> Add/2
  X0/1 -> Selector1/1, Selector2/1
  Selector1/1 -> dX/3
  Selector2/1 -> dV/3
  Rate Transition3/1 -> dV/2, dX/2, dA/2

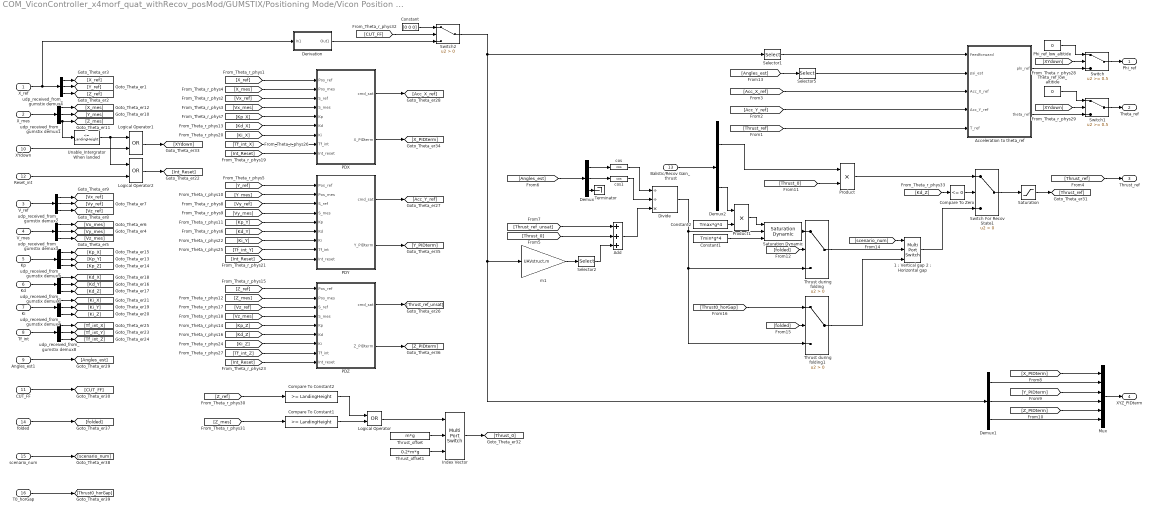
== system COM_ViconController_x4morf_quat_withRecov_posMod/GUMSTIX/Positioning Mode/Vicon Position  Controller/PositionController1 ==
  X_ref : Inport
  X_mes : Inport  Port=2
  V_ref : Inport  Port=3
  V_mes : Inport  Port=4
  Kp : Inport  Port=5
  Kd : Inport  Port=6
  Ki : Inport  Port=7
  Tf_int : Inport  Port=8
  Angles_est1 : Inport  Port=9
  XYdown : Inport  Port=10
  CUT_FF : Inport  Port=11
  Reset_int : Inport  Port=12
  Balistic/Recov Gain_thrust : Inport  Port=13
  folded : Inport  Port=14
  scenario_num : Inport  Port=15
  T0_horGap : Inport  Port=16
  "1 : Vertical gap 2 : Horizontal gap" : MultiPortSwitch  Inputs=2
  Acceleration to theta_ref : Subsystem
  Add : Sum  Inputs=+++
  Compare To Constant1 : simulink/Logic and Bit Operations/Compare To Constant  relop=>=  const=LandingHeight  OutDataTypeStr=uint8
  Compare To Constant2 : simulink/Logic and Bit Operations/Compare To Constant  relop=>=  const=LandingHeight  OutDataTypeStr=uint8
  Compare To Zero : simulink/Logic and Bit Operations/Compare To Zero  relop=<=  OutDataTypeStr=boolean
  Constant : Constant  Value=[0 0 0]  OutDataTypeStr=Inherit: Inherit via back propagation
  Constant1 : Constant  Value=Tmin*g*4  OutDataTypeStr=Inherit: Inherit via back propagation
  Constant2 : Constant  Value=Tmax*g*4  OutDataTypeStr=Inherit: Inherit via back propagation
  Demux : Demux  Outputs=3
  Demux1 : Demux  Outputs=3
  Demux2 : Demux  Outputs=2
  Derivation : Subsystem
  Divide : Product  Inputs=//*
  Index Vector : MultiPortSwitch  Inputs=2  DiagnosticForDefault=None
  Logical Operator : Logic  Operator=OR  AllPortsSameDT=off  OutDataTypeStr=boolean
  Logical Operator1 : Logic  Operator=OR  AllPortsSameDT=off  OutDataTypeStr=boolean
  Logical Operator2 : Logic  Operator=OR  AllPortsSameDT=off  OutDataTypeStr=boolean
  Mux : Mux  Inputs=[5 1 5 1 5 1]
  PDX : Subsystem  mask{Max_Sat=20*pi/180*9.81, Min_Sat=-20*pi/180*9.81}
  PDY : Subsystem  mask{Max_Sat=20*pi/180*9.81, Min_Sat=-20*pi/180*9.81}
  PDZ : Subsystem  mask{Max_Sat=Tmax*g*4, Min_Sat=Tmin*g*4}
  Phi_ref_low_altitide : Constant  Value=0  OutDataTypeStr=Inherit: Inherit via back propagation
  Product : Product
  Product1 : Product
  Saturation : Saturate  UpperLimit=Tmax*g*4  LowerLimit=Tmin*g*4
  Saturation Dynamic : simulink/Discontinuities/Saturation Dynamic  OutMin=[]  OutMax=[]  OutDataTypeStr=Inherit: Same as second input  OutDataType=fixdt(1, 16)  OutScaling=2^-10  DoSatur=off
  Selector1 : Selector  InputPortWidth=3  IndexOptions=Index vector (dialog)  Indices=[1 2]  OutputSizes=1
  Selector2 : Selector  InputPortWidth=3  IndexOptions=Index vector (dialog)  Indices=[3]  OutputSizes=1
  Selector5 : Selector  InputPortWidth=3  IndexOptions=Index vector (dialog)  Indices=[3]  OutputSizes=1
  Switch : Switch  Threshold=0.5
  Switch For Recov State1 : Switch  Criteria=u2 > Threshold
  Switch1 : Switch  Threshold=0.5
  Switch2 : Switch  Criteria=u2 > Threshold
  Terminator : Terminator
  Theta_ref_low_altitide : Constant  Value=0  OutDataTypeStr=Inherit: Inherit via back propagation
  Thrust during folding : Switch  Criteria=u2 > Threshold
  Thrust during folding1 : Switch  Criteria=u2 > Threshold
  Thrust_offset : Constant  Value=m*g  OutDataTypeStr=single  SampleTime=-1
  Thrust_offset1 : Constant  Value=0.2*m*g  OutDataTypeStr=single  SampleTime=-1
  Unable_Intergrator When landed : simulink/Logic and Bit Operations/Compare To Constant  relop=<=  const=LandingHeight  OutDataTypeStr=uint8
  cos : Trigonometry  Operator=cos
  cos1 : Trigonometry  Operator=cos
  m1 : Gain  Gain=UAVstruct.m
  udp_received_from_gumstix demux{1..8} (8 alike) : Demux  Outputs=[1 1 1]
  Phi_ref : Outport
  Theta_ref : Outport  Port=2
  Thrust_ref : Outport  Port=3
  XYZ_PIDterm : Outport  Port=4
  wires:
  udp_received_from_gumstix demux3/3 -> [Vz_mes]
  udp_received_from_gumstix demux3/2 -> [Vy_mes]
  udp_received_from_gumstix demux3/1 -> [Vx_mes]
  V_mes/1 -> udp_received_from_gumstix demux3/1
  udp_received_from_gumstix demux4/1 -> [X_ref]
  udp_received_from_gumstix demux4/2 -> [Y_ref]
  X_mes/1 -> udp_received_from_gumstix demux1/1
  udp_received_from_gumstix demux1/1 -> [X_mes]
  udp_received_from_gumstix demux1/2 -> [Y_mes]
  udp_received_from_gumstix demux1/3 -> [Z_mes], Unable_Intergrator When landed/1
  udp_received_from_gumstix demux2/3 -> [Vz_ref]
  udp_received_from_gumstix demux2/2 -> [Vy_ref]
  udp_received_from_gumstix demux2/1 -> [Vx_ref]
  V_ref/1 -> udp_received_from_gumstix demux2/1
  Kp/1 -> udp_received_from_gumstix demux5/1
  udp_received_from_gumstix demux5/3 -> [Kp_Z]
  udp_received_from_gumstix demux5/2 -> [Kp_Y]
  udp_received_from_gumstix demux5/1 -> [Kp_X]
  Kd/1 -> udp_received_from_gumstix demux6/1
  udp_received_from_gumstix demux6/3 -> [Kd_Z]
  udp_received_from_gumstix demux6/2 -> [Kd_Y]
  udp_received_from_gumstix demux6/1 -> [Kd_X]
  udp_received_from_gumstix demux4/3 -> [Z_ref]
  udp_received_from_gumstix demux7/3 -> [Ki_Z]
  udp_received_from_gumstix demux7/2 -> [Ki_Y]
  udp_received_from_gumstix demux7/1 -> [Ki_X]
  Ki/1 -> udp_received_from_gumstix demux7/1
  udp_received_from_gumstix demux8/3 -> [Tf_int_Z]
  udp_received_from_gumstix demux8/2 -> [Tf_int_Y]
  udp_received_from_gumstix demux8/1 -> [Tf_int_X]
  Tf_int/1 -> udp_received_from_gumstix demux8/1
  Acceleration to theta_ref/1(phi_ref) -> Switch/3
  [XYdown] -> Switch/2
  [XYdown] -> Switch1/2
  Acceleration to theta_ref/2(theta_ref) -> Switch1/3
  Switch1/1 -> Theta_ref/1
  Switch/1 -> Phi_ref/1
  Phi_ref_low_altitide/1 -> Switch/1
  Theta_ref_low_altitide/1 -> Switch1/1
  [Acc_X_ref] -> Acceleration to theta_ref/3(Acc_X_ref)
  [Acc_Y_ref] -> Acceleration to theta_ref/4(Acc_Y_ref)
  [Thrust_ref] -> Thrust_ref/1
  [Thrust_ref] -> Acceleration to theta_ref/5(T_ref)
  Selector5/1 -> Acceleration to theta_ref/2(psi_est)
  [Angles_est] -> Selector5/1
  Angles_est1/1 -> [Angles_est]
  [Thrust_0] -> Add/2
  [Angles_est] -> Demux/1
  Demux/3 -> Terminator/1
  Demux/1 -> cos/1
  Demux/2 -> cos1/1
  cos/1 -> Divide/1
  cos1/1 -> Divide/2
  [Thrust_ref_unsat] -> Add/1
  Add/1 -> Divide/3
  Selector2/1 -> Add/3
  Selector1/1 -> Acceleration to theta_ref/1(Feedforward)
  Saturation/1 -> [Thrust_ref]
  X_ref/1 -> Derivation/1(In1), udp_received_from_gumstix demux4/1
  m1/1 -> Selector2/1
  Thrust_offset/1 -> Index Vector/2
  Thrust_offset1/1 -> Index Vector/3
  Logical Operator/1 -> Index Vector/1
  Compare To Constant1/1 -> Logical Operator/2
  Compare To Constant2/1 -> Logical Operator/1
  [Z_mes] -> Compare To Constant1/1
  [Z_ref] -> Compare To Constant2/1
  Index Vector/1 -> [Thrust_0]
  Unable_Intergrator When landed/1 -> Logical Operator2/1, Logical Operator1/1
  XYdown/1 -> Logical Operator1/2
  Logical Operator1/1 -> [XYdown]
  CUT_FF/1 -> [CUT_FF]
  [CUT_FF] -> Switch2/2
  Derivation/1(Out1) -> Switch2/3
  Switch2/1 -> Selector1/1, Demux1/1, m1/1
  Constant/1 -> Switch2/1
  Logical Operator2/1 -> [Int_Reset]
  Reset_int/1 -> Logical Operator2/2
  [X_ref] -> PDX/1(Pos_ref)
  [X_mes] -> PDX/2(Pos_mes)
  [Kp_X] -> PDX/5(Kp)
  [Kd_X] -> PDX/6(Kd)
  [Vx_mes] -> PDX/4(S_mes)
  [Y_ref] -> PDY/1(Pos_ref)
  [Y_mes] -> PDY/2(Pos_mes)
  [Kp_Y] -> PDY/5(Kp)
  [Kd_Y] -> PDY/6(Kd)
  [Vy_ref] -> PDY/3(S_ref)
  [Vy_mes] -> PDY/4(S_mes)
  [Vx_ref] -> PDX/3(S_ref)
  [Ki_X] -> PDX/7(Ki)
  [Ki_Y] -> PDY/7(Ki)
  [Int_Reset] -> PDY/9(Int_reset)
  [Z_ref] -> PDZ/1(Pos_ref)
  [Z_mes] -> PDZ/2(Pos_mes)
  [Vz_ref] -> PDZ/3(S_ref)
  [Vz_mes] -> PDZ/4(S_mes)
  [Kp_Z] -> PDZ/5(Kp)
  [Kd_Z] -> PDZ/6(Kd)
  [Ki_Z] -> PDZ/7(Ki)
  [Tf_int_Y] -> PDY/8(Tf_int)
  [Tf_int_X] -> PDX/8(Tf_int)
  [Int_Reset] -> PDX/9(Int_reset)
  [Tf_int_Z] -> PDZ/8(Tf_int)
  [Int_Reset] -> PDZ/9(Int_reset)
  PDY/1(cmd_sat) -> [Acc_Y_ref]
  PDX/1(cmd_sat) -> [Acc_X_ref]
  PDZ/1(cmd_sat) -> [Thrust_ref_unsat]
  PDX/2(X_PIDterm) -> [X_PIDterm]
  PDY/2(Y_PIDterm) -> [Y_PIDterm]
  PDZ/2(Z_PIDterm) -> [Z_PIDterm]
  [Y_PIDterm] -> Mux/3
  Mux/1 -> XYZ_PIDterm/1
  [X_PIDterm] -> Mux/1
  [Z_PIDterm] -> Mux/5
  [Kd_Z] -> Compare To Zero/1
  Compare To Zero/1 -> Switch For Recov State1/2
  Switch For Recov State1/1 -> Saturation/1
  [Thrust_0] -> Product/2
  Product/1 -> Switch For Recov State1/1
  Demux1/1 -> Mux/2
  Demux1/2 -> Mux/4
  Demux1/3 -> Mux/6
  folded/1 -> [folded]
  [folded] -> Thrust during folding/2
  Saturation Dynamic/1 -> Thrust during folding/1
  Divide/1 -> Saturation Dynamic/2, Thrust during folding1/3, Thrust during folding/3
  Constant1/1 -> Saturation Dynamic/3
  Product1/1 -> Saturation Dynamic/1
  Constant2/1 -> Product1/2
  Balistic/Recov Gain_thrust/1 -> Demux2/1
  Demux2/1 -> Product/1
  Demux2/2 -> Product1/1
  scenario_num/1 -> [scenario_num]
  Thrust during folding/1 -> "1 : Vertical gap 2 : Horizontal gap"/2
  [folded] -> Thrust during folding1/2
  "1 : Vertical gap 2 : Horizontal gap"/1 -> Switch For Recov State1/3
  T0_horGap/1 -> [Thrust0_horGap]
  [Thrust0_horGap] -> Thrust during folding1/1
  Thrust during folding1/1 -> "1 : Vertical gap 2 : Horizontal gap"/3
  [scenario_num] -> "1 : Vertical gap 2 : Horizontal gap"/1

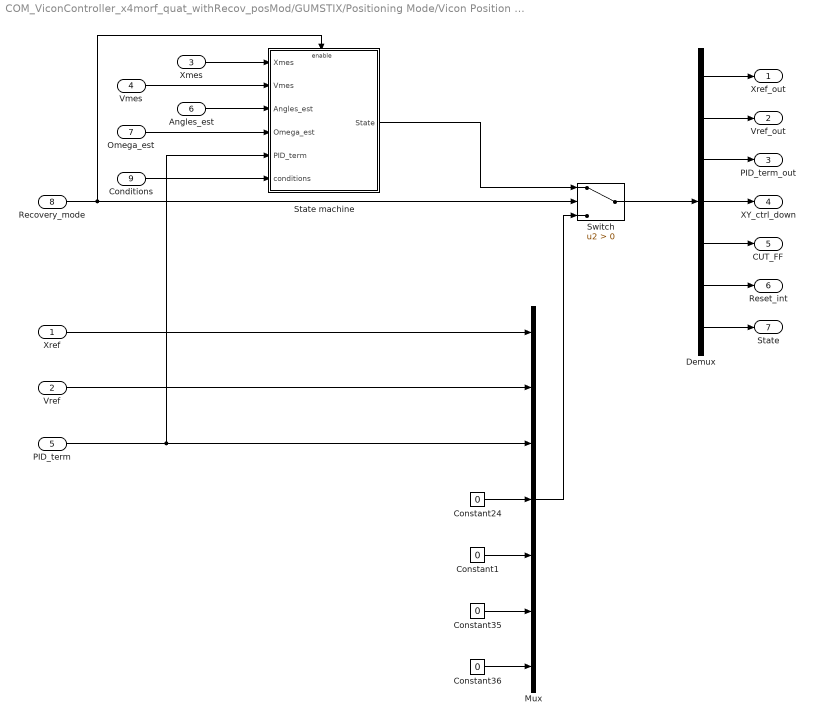
== system COM_ViconController_x4morf_quat_withRecov_posMod/GUMSTIX/Positioning Mode/Vicon Position  Controller/Recovery state machine ==
  Xref : Inport
  Vref : Inport  Port=2
  Xmes : Inport  Port=3
  Vmes : Inport  Port=4
  PID_term : Inport  Port=5
  Angles_est : Inport  Port=6
  Omega_est : Inport  Port=7
  Recovery_mode : Inport  Port=8
  Conditions : Inport  Port=9
  Constant{1,24,35..36} (4 alike) : Constant  Value=0  OutDataTypeStr=Inherit: Inherit via back propagation
  Demux : Demux  Outputs=[3 3 12 1 1 1 1]
  Mux : Mux  Inputs=7
  State machine : Subsystem
  Switch : Switch  Criteria=u2 > Threshold
  Xref_out : Outport
  Vref_out : Outport  Port=2
  PID_term_out : Outport  Port=3
  XY_ctrl_down : Outport  Port=4
  CUT_FF : Outport  Port=5
  Reset_int : Outport  Port=6
  State : Outport  Port=7
  wires:
  Demux/1 -> Xref_out/1
  Demux/2 -> Vref_out/1
  Demux/3 -> PID_term_out/1
  Demux/4 -> XY_ctrl_down/1
  Demux/5 -> CUT_FF/1
  Xref/1 -> Mux/1
  Vref/1 -> Mux/2
  Constant24/1 -> Mux/4
  Constant1/1 -> Mux/5
  Mux/1 -> Switch/3
  Vmes/1 -> State machine/2(Vmes)
  Demux/6 -> Reset_int/1
  Constant35/1 -> Mux/6
  PID_term/1 -> State machine/5(PID_term), Mux/3
  Switch/1 -> Demux/1
  Demux/7 -> State/1
  Constant36/1 -> Mux/7
  Recovery_mode/1 -> Switch/2, State machine/Enable
  State machine/1(State) -> Switch/1
  Angles_est/1 -> State machine/3(Angles_est)
  Omega_est/1 -> State machine/4(Omega_est)
  Xmes/1 -> State machine/1(Xmes)
  Conditions/1 -> State machine/6(conditions)

== system COM_ViconController_x4morf_quat_withRecov_posMod/GUMSTIX/Attitude controller/CTL_ATT_NL/Angles Disturbances/Triggered Subsystem ==
  AnglesDist Mag : Inport
  Dt : Inport  Port=2
  Enable : EnablePort  StatesWhenEnabling=reset
  Constant : Constant  OutDataTypeStr=single
  Discrete-Time Integrator : DiscreteIntegrator  SampleTime=-1  ICPrevOutput=DiscIntNeverNeededParam  ICPrevScaledInput=DiscIntNeverNeededParam
  MATLAB Function : MATLAB Function  TreatAsAtomicUnit=on
  DisturbAngles : Outport  InitialOutput=[0 0 0]
  wires:
  AnglesDist Mag/1 -> MATLAB Function/1(AnglesDistMag)
  Constant/1 -> Discrete-Time Integrator/1
  Discrete-Time Integrator/1 -> MATLAB Function/2(Time)
  Dt/1 -> MATLAB Function/3(Dt)
  MATLAB Function/1(AnglesDist) -> DisturbAngles/1

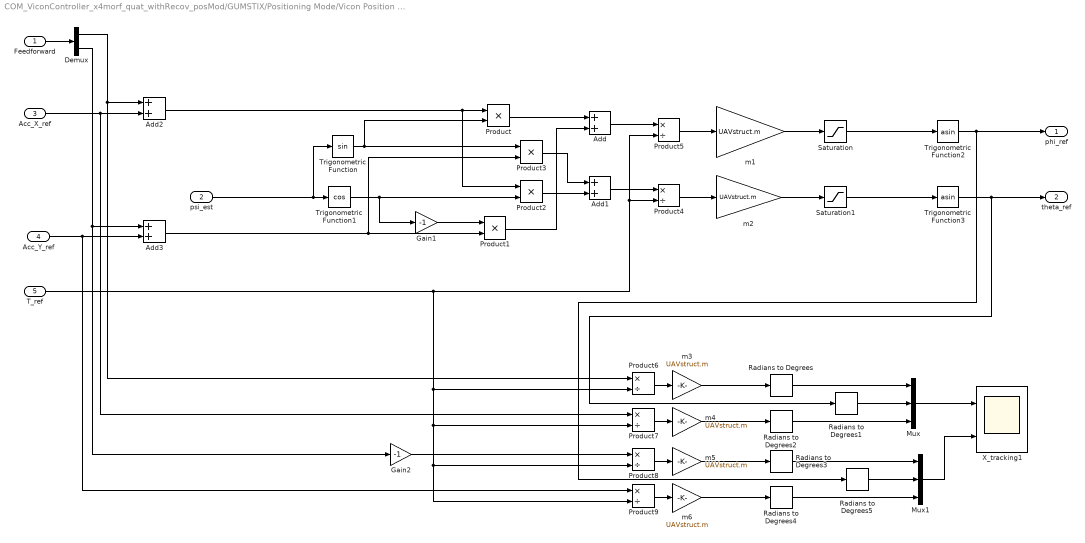
== system COM_ViconController_x4morf_quat_withRecov_posMod/GUMSTIX/Positioning Mode/Vicon Position  Controller/PositionController1/Acceleration to theta_ref ==
  Feedforward : Inport
  psi_est : Inport  Port=2
  Acc_X_ref : Inport  Port=3
  Acc_Y_ref : Inport  Port=4
  T_ref : Inport  Port=5
  Add{,1..3} (4 alike) : Sum
  Demux : Demux  Outputs=2
  Gain1 : Gain  Gain=-1
  Gain2 : Gain  Gain=-1
  Mux : Mux  Inputs=3
  Mux1 : Mux  Inputs=3
  Product{,1..3} (4 alike) : Product  RndMeth=Zero
  Product{4..9} (6 alike) : Product  Inputs=*/  RndMeth=Zero
  Radians to Degrees{,1..5} (6 alike) : simulink_extras/Transformations/Radians to Degrees
  Saturation : Saturate  UpperLimit=sin(45*pi/180)  LowerLimit=sin(-45*pi/180)
  Saturation1 : Saturate  UpperLimit=sin(45*pi/180)  LowerLimit=sin(-45*pi/180)
  Trigonometric Function : Trigonometry
  Trigonometric Function1 : Trigonometry  Operator=cos
  Trigonometric Function2 : Trigonometry  Operator=asin
  Trigonometric Function3 : Trigonometry  Operator=asin
  X_tracking1 : Scope  NumInputPorts=2
  m{1..6} (6 alike) : Gain  Gain=UAVstruct.m
  phi_ref : Outport
  theta_ref : Outport  Port=2
  wires:
  psi_est/1 -> Trigonometric Function/1, Trigonometric Function1/1
  Trigonometric Function/1 -> Product3/1, Product/2
  Trigonometric Function1/1 -> Product2/2, Gain1/1
  Product1/1 -> Add/2
  Product/1 -> Add/1
  Product3/1 -> Add1/1
  Product2/1 -> Add1/2
  Acc_X_ref/1 -> Add2/2, Product7/1
  Demux/1 -> Add2/1, Product6/1
  Demux/2 -> Add3/1, Gain2/1
  Acc_Y_ref/1 -> Add3/2, Product9/1
  Add2/1 -> Product2/1, Product/1
  Add3/1 -> Product3/2, Product1/2
  Product5/1 -> m1/1
  m1/1 -> Saturation/1
  Add/1 -> Product5/1
  Trigonometric Function2/1 -> phi_ref/1, Radians to Degrees5/1
  Product4/1 -> m2/1
  m2/1 -> Saturation1/1
  Trigonometric Function3/1 -> theta_ref/1, Radians to Degrees1/1
  Add1/1 -> Product4/1
  T_ref/1 -> Product4/2, Product5/2, Product6/2, Product7/2, Product8/2, Product9/2
  Saturation/1 -> Trigonometric Function2/1
  Saturation1/1 -> Trigonometric Function3/1
  Gain1/1 -> Product1/1
  Radians to Degrees/1 -> Mux/1
  Radians to Degrees1/1 -> Mux/2
  Product6/1 -> m3/1
  m3/1 -> Radians to Degrees/1
  Product7/1 -> m4/1
  m4/1 -> Radians to Degrees2/1
  Radians to Degrees2/1 -> Mux/3
  Mux/1 -> X_tracking1/1
  Mux1/1 -> X_tracking1/2
  Product8/1 -> m5/1
  m5/1 -> Radians to Degrees3/1
  Radians to Degrees3/1 -> Mux1/1
  Radians to Degrees4/1 -> Mux1/3
  Product9/1 -> m6/1
  m6/1 -> Radians to Degrees4/1
  Radians to Degrees5/1 -> Mux1/2
  Gain2/1 -> Product8/1
  Feedforward/1 -> Demux/1

== system COM_ViconController_x4morf_quat_withRecov_posMod/GUMSTIX/Positioning Mode/Vicon Position  Controller/PositionController1/Derivation ==
  In1 : Inport
  Demux : Demux  Outputs=3
  Discrete Derivative : simulink/Discrete/Discrete Derivative  gainval=1.0  ICPrevScaledInput=Velocity_0(1)  InputProcessing=Inherited  OutMin=[]  OutMax=[]  OutDataType=fixdt(1, 16)  OutScaling=2^-10  DoSatur=off
  Discrete Derivative1 : simulink/Discrete/Discrete Derivative  gainval=1.0  ICPrevScaledInput=Velocity_0(2)  InputProcessing=Inherited  OutMin=[]  OutMax=[]  OutDataType=fixdt(1, 16)  OutScaling=2^-10  DoSatur=off
  Discrete Derivative2 : simulink/Discrete/Discrete Derivative  gainval=1.0  ICPrevScaledInput=Velocity_0(3)  InputProcessing=Inherited  OutMin=[]  OutMax=[]  OutDataType=fixdt(1, 16)  OutScaling=2^-10  DoSatur=off
  Discrete Derivative3 : simulink/Discrete/Discrete Derivative  gainval=1.0  ICPrevScaledInput=0  InputProcessing=Inherited  OutMin=[]  OutMax=[]  OutDataType=fixdt(1, 16)  OutScaling=2^-10  DoSatur=off
  Discrete Derivative4 : simulink/Discrete/Discrete Derivative  gainval=1.0  ICPrevScaledInput=0  InputProcessing=Inherited  OutMin=[]  OutMax=[]  OutDataType=fixdt(1, 16)  OutScaling=2^-10  DoSatur=off
  Discrete Derivative5 : simulink/Discrete/Discrete Derivative  gainval=1.0  ICPrevScaledInput=0  InputProcessing=Inherited  OutMin=[]  OutMax=[]  OutDataType=fixdt(1, 16)  OutScaling=2^-10  DoSatur=off
  Mux : Mux  Inputs=3
  Out1 : Outport
  wires:
  In1/1 -> Demux/1
  Mux/1 -> Out1/1
  Demux/1 -> Discrete Derivative/1
  Discrete Derivative/1 -> Discrete Derivative3/1
  Demux/2 -> Discrete Derivative1/1
  Discrete Derivative1/1 -> Discrete Derivative4/1
  Demux/3 -> Discrete Derivative2/1
  Discrete Derivative2/1 -> Discrete Derivative5/1
  Discrete Derivative3/1 -> Mux/1
  Discrete Derivative4/1 -> Mux/2
  Discrete Derivative5/1 -> Mux/3
